simulink library "StopConditionsBlock"  (R2018b)
settings: Solver=VariableStepAuto  StartTime=0.0  StopTime=10.0  RelTol=1e-3
undefined symbols (not defined in the file): stop_altitude_ft, stop_range_ft
settings Model: Creator=BI28030  LastModifiedBy=BI28030

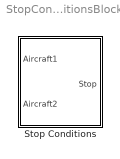
== system StopConditionsBlock ==
  Stop Conditions : Subsystem  mask(StopConditions){range_limit_ft=stop_range_ft, altitude_limit_ft=stop_altitude_ft}
      mask prompts: range_limit_ft "Stop range (ft)"; altitude_limit_ft "Stop altitude (ft)"
      mask help:
      | Returns non-zero once the relative location of two aircraft have been within and then outside a cylinder of the specified radius and height.
      |
      | The class StopConditions can be used to programmatically set the parameters of Stop Conditions blocks.
      mask Help:
      | Returns non-zero once the relative location of two aircraft have been within
      | and then outside a cylinder of the specified radius and height.
      | 
      | INPUTS
      | ==========
      | Aircraft1 - A CASSATT v6 AircraftState bus from first aircraft
      | Aircraft2 - A CASSATT v6 AircraftState bus from second aircraft
      | 
      | OUTPUTS
      | ==========
      | Stop - non-zero once stop conditions have been met, otherwise zero
      | 
      | PARAMETERS
      | ==========
      | range_limit_ft - Stopping horizontal range in feet
      | altitude_limit_ft - Stopping vertical separation in feet
      | 
      | The class StopConditions can be used to programmatically set the parameters of Stop Conditions blocks.

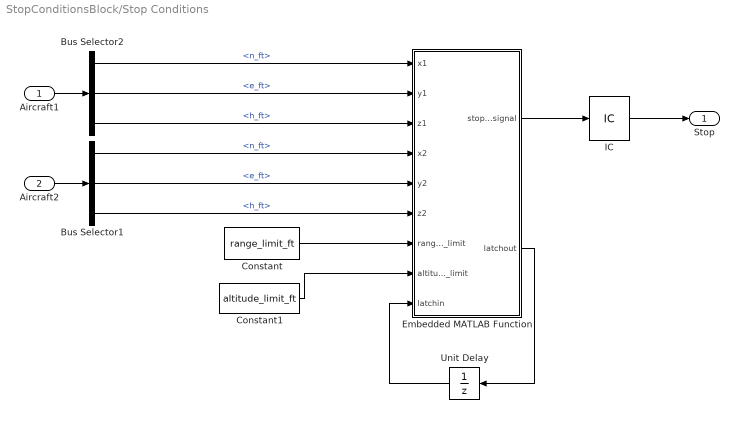
== system StopConditionsBlock/Stop Conditions ==
  Aircraft1 : Inport  OutDataTypeStr=Bus: AircraftState
  Aircraft2 : Inport  Port=2  OutDataTypeStr=Bus: AircraftState
  Bus Selector1 : BusSelector  OutputSignals=n_ft,e_ft,h_ft
  Bus Selector2 : BusSelector  OutputSignals=n_ft,e_ft,h_ft
  Constant : Constant  Value=range_limit_ft
  Constant1 : Constant  Value=altitude_limit_ft
  Embedded MATLAB Function : MATLAB Function  TreatAsAtomicUnit=on
  IC : InitialCondition  Value=0
  Unit Delay : UnitDelay  SampleTime=-1
  Stop : Outport
  wires:
  Embedded MATLAB Function/1(stop_signal) -> IC/1
  Aircraft1/1 -> Bus Selector2/1
  Aircraft2/1 -> Bus Selector1/1
  Bus Selector2/1 -> Embedded MATLAB Function/1(x1)  "<n_ft>"
  Bus Selector2/2 -> Embedded MATLAB Function/2(y1)  "<e_ft>"
  Bus Selector1/1 -> Embedded MATLAB Function/4(x2)  "<n_ft>"
  Bus Selector1/2 -> Embedded MATLAB Function/5(y2)  "<e_ft>"
  Bus Selector1/3 -> Embedded MATLAB Function/6(z2)  "<h_ft>"
  Bus Selector2/3 -> Embedded MATLAB Function/3(z1)  "<h_ft>"
  Constant/1 -> Embedded MATLAB Function/7(range_limit)
  Constant1/1 -> Embedded MATLAB Function/8(altitude_limit)
  IC/1 -> Stop/1
  Embedded MATLAB Function/2(latchout) -> Unit Delay/1
  Unit Delay/1 -> Embedded MATLAB Function/9(latchin)

== matlab function StopConditionsBlock/Stop Conditions/Embedded MATLAB Function ==
  data: x1 input; y1 input; z1 input; x2 input; y2 input; z2 input; stop_signal output; range_limit input =9999; altitude_limit input =1e6; latchin input; latchout output
function [stop_signal,latchout] = fcn(x1, y1, z1, x2, y2, z2, range_limit, altitude_limit, latchin)
% This block supports an embeddable subset of the MATLAB language.
% See the help menu for details. 
% Latch will ensure that will not exit simulation due to exiting cylinder unless have entered cylinder first

range2 = ((x1-x2)^2 + (y1-y2)^2);  % range-squared
rel_altitude = abs(z1-z2);

latchout = latchin;

stop_signal = 0;
if ((range2 > (range_limit^2) || rel_altitude > altitude_limit)) && latchin==1
    stop_signal = 1;
elseif ((range2 < (range_limit^2) && rel_altitude < altitude_limit)) && latchin==0
    latchout=1;
end
